simulink model "Taller4_Bloques"  (R2024a)
settings: Solver=ode4  StartTime=0.0  StopTime=0.015  RelTol=1e-3
values from neighbouring files (symbols this model uses):
  A1 = [-R/L -1/L; 1/Cap 0]    [Taller4.m]
  B1 = [1/L; 0]    [Taller4.m]
  C1 = [0 1; 1 0]    [Taller4.m]
settings Model: Creator=UsuarioF  LastModifiedBy=UsuarioF

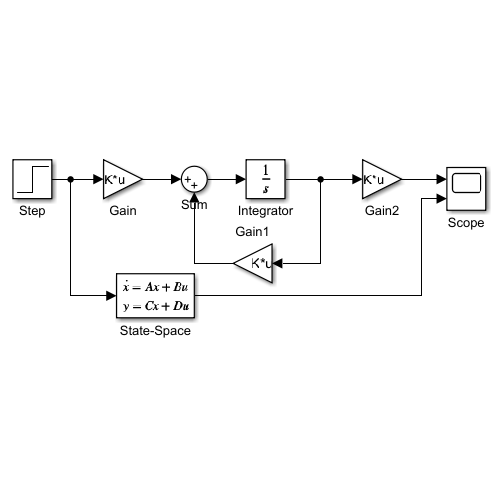
[thumbnail: Simulink's stored preview of the top-level diagram]
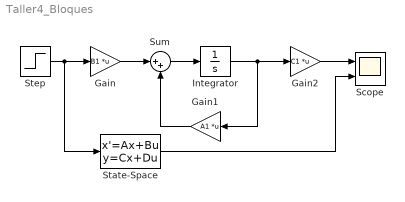
== system Taller4_Bloques ==
  Gain : Gain  Gain=B1  Multiplication=Matrix(K*u)
  Gain1 : Gain  Gain=A1  Multiplication=Matrix(K*u)
  Gain2 : Gain  Gain=C1  Multiplication=Matrix(K*u)
  Integrator : Integrator
  Scope : Scope  NumInputPorts=2
  State-Space : StateSpace  A=A1  B=B1  C=C1  D=[0; 0]  InitialCondition=0
  Step : Step  Time=0.01  SampleTime=0
  Sum : Sum  Inputs=|++
  wires:
  Gain/1 -> Sum/1
  Step/1 -> State-Space/1, Gain/1
  Gain1/1 -> Sum/2
  Sum/1 -> Integrator/1
  Integrator/1 -> Gain2/1, Gain1/1
  Gain2/1 -> Scope/1
  State-Space/1 -> Scope/2
